simulink model "MON_sl_after_harness"  (R2016a)
settings: Solver=FixedStepDiscrete  StartTime=0  StopTime=0.01  FixedStep=0.01  RelTol=1e-3
undefined symbols (not defined in the file or in its folder): dt, sigbuilder_block
libraries: simulink x1
settings Model: SldvGeneratedHarnessModel=TestUnitModel=MON_sl_after|  MBDTemplateVer=1.1  ModelType=Feature  LastModifiedBy=jdbackes
settings DataIOCC: LimitDataPoints=on  SaveFormat=StructureWithTime
settings OptimizationCC: BlockReduction=off  ExpressionFolding=off
settings DebuggingCC: InheritedTsInSrcMsg=none  AllowSymbolicDim=off
settings ModelReferenceCC: PropagateSignalLabelsOutOfModel=off
settings RTWCC: Description=Generic Real-Time Target
settings GRTTargetCC: GeneratePreprocessorConditionals=Use local settings
settings ConfigComp: DVMode=PropertyProving  DVTestSuiteOptimization=CombinedObjectives (Nonlinear Extended)  DVAssertions=EnableAll  DVProofAssumptions=EnableAll  DVDisplayReport=off

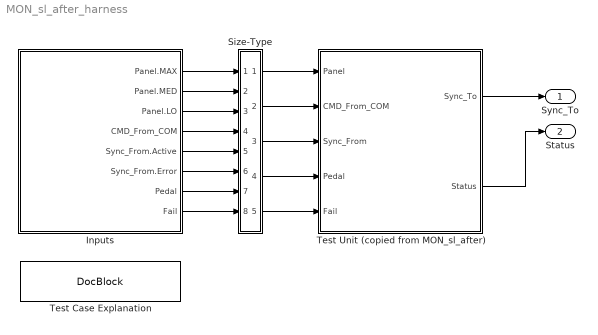
== system MON_sl_after_harness ==
  Inputs : Subsystem  Tag=STV Subsys  LoadFcn=sigbuilder_block('load',[50 50 520 400 ]);  StartFcn=sigbuilder_block('start');  StopFcn=sigbuilder_block('stop');  ClipboardFcn=sigbuilder_block('clipboard');  mask(Sigbuilder block){}
      mask init:
      | if ~strcmp(get_param(bdroot(gcb),'SimulationStatus'),'stopped'),tuvar = sigbuilder_block('maskInit'); end
      settings: CopyFcn=sigbuilder_block('copy');  DeleteFcn=sigbuilder_block('delete');  ModelCloseFcn=sigbuilder_block('modelClose');  PreSaveFcn=sigbuilder_block('preSave');  PauseFcn=sigbuilder_block('pause');  ContinueFcn=sigbuilder_block('continue');  NameChangeFcn=sigbuilder_block('namechange');  OpenFcn=sigbuilder_block('open');  CloseFcn=sigbuilder_block('close');
      mask Display: plot(0, 0, 100, 100,[2, 2, 32, 32, 2], [68, 8, 8, 68, 68],[32, 2], [38, 38], [32, 19, 2],[53, 60, 44], [32, 17, 17, 2],[16, 16, 31, 31]);txt = getActiveGroup(gcbh);text(2, 100, txt,'verticalAlignment', 'top');
  Size-Type : Subsystem
  Test Case Explanation : simulink/Model-Wide Utilities/DocBlock  DocumentType=Text
  Test Unit (copied from MON_sl_after) : Subsystem
  Sync_To : Outport  OutDataTypeStr=Bus: SyncMsgImpl  BusOutputAsStruct=on
  Status : Outport  Port=2  OutDataTypeStr=Bus: ChannelStatusImpl  BusOutputAsStruct=on
  wires:
  Inputs/1(Panel.MAX) -> Size-Type/1(In1)
  Inputs/2(Panel.MED) -> Size-Type/2(In2)
  Inputs/3(Panel.LO) -> Size-Type/3(In3)
  Size-Type/1(Out1) -> Test Unit (copied from MON_sl_after)/1(Panel)
  Inputs/4(CMD_From_COM) -> Size-Type/4(In4)
  Size-Type/2(Out2) -> Test Unit (copied from MON_sl_after)/2(CMD_From_COM)
  Inputs/5(Sync_From.Active) -> Size-Type/5(In5)
  Inputs/6(Sync_From.Error) -> Size-Type/6(In6)
  Size-Type/3(Out3) -> Test Unit (copied from MON_sl_after)/3(Sync_From)
  Inputs/7(Pedal) -> Size-Type/7(In7)
  Size-Type/4(Out4) -> Test Unit (copied from MON_sl_after)/4(Pedal)
  Inputs/8(Fail) -> Size-Type/8(In8)
  Size-Type/5(Out5) -> Test Unit (copied from MON_sl_after)/5(Fail)
  Test Unit (copied from MON_sl_after)/1(Sync_To) -> Sync_To/1
  Test Unit (copied from MON_sl_after)/2(Status) -> Status/1

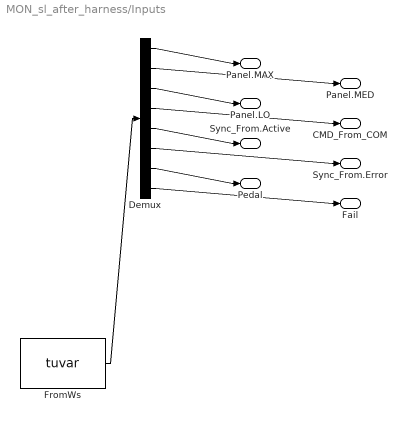
== system MON_sl_after_harness/Inputs ==
  Demux : Demux  Tag=STV Demux  Outputs=8
  FromWs : FromWorkspace  Tag=STV FromWs  VariableName=tuvar  SampleTime=0
      SigBuilderData=|
      | dataSet.timeRange = [0 0.01]
      | dataSet.name = 'Counterexample 1'
      | sbobj.Name = 'Signal Builder'
      | sbobj.Groups.Name = 'Counterexample 1'
      | sbobj.Groups.Signals(1).Name = 'Panel.MAX'
      | sbobj.Groups.Signals(1).XData = [0 0.01]
      | sbobj.Groups.Signals(1).YData = [0 0]
      | sbobj.Groups.Signals(2).Name = 'Panel.MED'
      | sbobj.Groups.Signals(2).XData = [0 0.01]
      | sbobj.Groups.Signals(2).YData = [0 0]
      | sbobj.Groups.Signals(3).Name = 'Panel.LO'
      | sbobj.Groups.Signals(3).XData = [0 0.01]
      | sbobj.Groups.Signals(3).YData = [1 1]
      | sbobj.Groups.Signals(4).Name = 'CMD_From_COM'
      | sbobj.Groups.Signals(4).XData = [0 0.01]
      | sbobj.Groups.Signals(4).YData = [1567609200 1567609200]
      | sbobj.Groups.Signals(5).Name = 'Sync_From.Active'
      | sbobj.Groups.Signals(5).XData = [0 0.01]
      | sbobj.Groups.Signals(5).YData = [1 1]
      | sbobj.Groups.Signals(6).Name = 'Sync_From.Error'
      | sbobj.Groups.Signals(6).XData = [0 0.01]
      | sbobj.Groups.Signals(6).YData = [1 1]
      | sbobj.Groups.Signals(7).Name = 'Pedal'
      | sbobj.Groups.Signals(7).XData = [0 0.01]
      | sbobj.Groups.Signals(7).YData = [1801054272 1801054272]
      | sbobj.Groups.Signals(8).Name = 'Fail'
      | sbobj.Groups.Signals(8).XData = [0 0.01]
      | sbobj.Groups.Signals(8).YData = [0 0]
      | sbobj.Groups.TimeRange = [0 0.01]
  Panel.MAX : Outport  Tag=STV Outport
  Panel.MED : Outport  Tag=STV Outport  Port=2
  Panel.LO : Outport  Tag=STV Outport  Port=3
  CMD_From_COM : Outport  Tag=STV Outport  Port=4
  Sync_From.Active : Outport  Tag=STV Outport  Port=5
  Sync_From.Error : Outport  Tag=STV Outport  Port=6
  Pedal : Outport  Tag=STV Outport  Port=7
  Fail : Outport  Tag=STV Outport  Port=8
  wires:
  FromWs/1 -> Demux/1
  Demux/1 -> Panel.MAX/1
  Demux/2 -> Panel.MED/1
  Demux/3 -> Panel.LO/1
  Demux/4 -> CMD_From_COM/1
  Demux/5 -> Sync_From.Active/1
  Demux/6 -> Sync_From.Error/1
  Demux/7 -> Pedal/1
  Demux/8 -> Fail/1

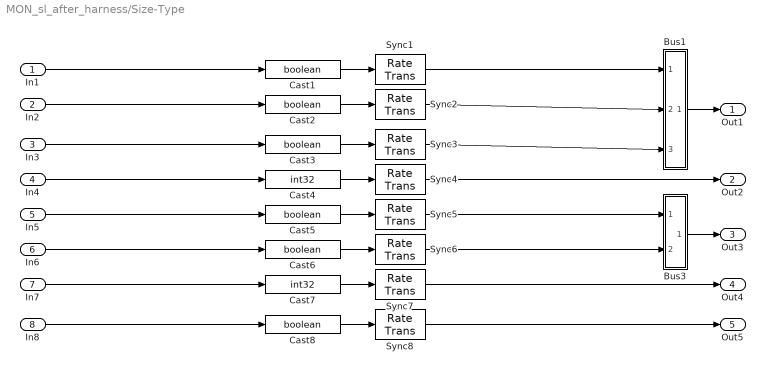
== system MON_sl_after_harness/Size-Type ==
  In1 : Inport
  In2 : Inport  Port=2
  In3 : Inport  Port=3
  In4 : Inport  Port=4
  In5 : Inport  Port=5
  In6 : Inport  Port=6
  In7 : Inport  Port=7
  In8 : Inport  Port=8
  Bus1 : Subsystem
  Bus3 : Subsystem
  Cast{1..3,5..6,8} (6 alike) : DataTypeConversion  OutDataTypeStr=boolean  RndMeth=Nearest  SaturateOnIntegerOverflow=on
  Cast4 : DataTypeConversion  OutDataTypeStr=int32  RndMeth=Nearest  SaturateOnIntegerOverflow=on
  Cast7 : DataTypeConversion  OutDataTypeStr=int32  RndMeth=Nearest  SaturateOnIntegerOverflow=on
  Sync{1..8} (8 alike) : RateTransition  OutPortSampleTime=[0.01,0]
  Out1 : Outport
  Out2 : Outport  Port=2
  Out3 : Outport  Port=3
  Out4 : Outport  Port=4
  Out5 : Outport  Port=5
  wires:
  In1/1 -> Cast1/1
  Cast1/1 -> Sync1/1
  In2/1 -> Cast2/1
  Cast2/1 -> Sync2/1
  In3/1 -> Cast3/1
  Cast3/1 -> Sync3/1
  Sync1/1 -> Bus1/1(Panel(1).MAX)
  Sync2/1 -> Bus1/2(Panel(1).MED)
  Sync3/1 -> Bus1/3(Panel(1).LO)
  Bus1/1(Out) -> Out1/1
  In4/1 -> Cast4/1
  Cast4/1 -> Sync4/1
  Sync4/1 -> Out2/1
  In5/1 -> Cast5/1
  Cast5/1 -> Sync5/1
  In6/1 -> Cast6/1
  Cast6/1 -> Sync6/1
  Sync5/1 -> Bus3/1(Sync_From(1).Active)
  Sync6/1 -> Bus3/2(Sync_From(1).Error)
  Bus3/1(Out) -> Out3/1
  In7/1 -> Cast7/1
  Cast7/1 -> Sync7/1
  Sync7/1 -> Out4/1
  In8/1 -> Cast8/1
  Cast8/1 -> Sync8/1
  Sync8/1 -> Out5/1

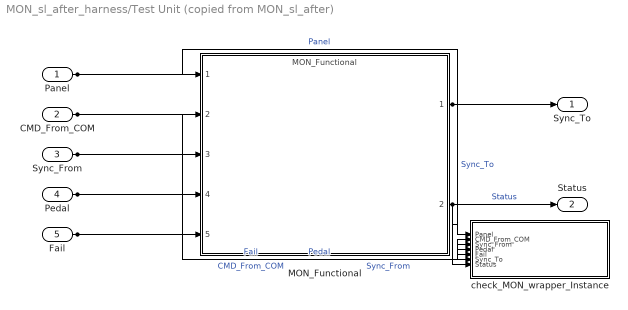
== system MON_sl_after_harness/Test Unit (copied from MON_sl_after) ==
  Panel : Inport  OutDataTypeStr=Bus: PanelMsgImpl  SampleTime=dt  Interpolate=off  BusOutputAsStruct=on
  CMD_From_COM : Inport  Port=2  OutDataTypeStr=int32  SampleTime=dt  Interpolate=off
  Sync_From : Inport  Port=3  OutDataTypeStr=Bus: SyncMsgImpl  SampleTime=dt  Interpolate=off  BusOutputAsStruct=on
  Pedal : Inport  Port=4  OutDataTypeStr=int32  SampleTime=dt  Interpolate=off
  Fail : Inport  Port=5  OutDataTypeStr=boolean  SampleTime=dt  Interpolate=off
  MON_Functional : ModelReference  ModelNameDialog=MON_Functional.slx  SimulationMode=Normal  ModelReferenceVersion=1.2
  check_MON_wrapper_Instance : MATLAB Function  TreatAsAtomicUnit=on  mask(VerificationSubsystem){}
  Sync_To : Outport  OutDataTypeStr=Bus: SyncMsgImpl  BusOutputAsStruct=on
  Status : Outport  Port=2  OutDataTypeStr=Bus: ChannelStatusImpl  BusOutputAsStruct=on
  wires:
  MON_Functional/1 -> check_MON_wrapper_Instance/6(Sync_To), Sync_To/1  "Sync_To"
  MON_Functional/2 -> check_MON_wrapper_Instance/7(Status), Status/1  "Status"
  Panel/1 -> check_MON_wrapper_Instance/1(Panel), MON_Functional/1  "Panel"
  CMD_From_COM/1 -> check_MON_wrapper_Instance/2(CMD_From_COM), MON_Functional/2  "CMD_From_COM"
  Sync_From/1 -> check_MON_wrapper_Instance/3(Sync_From), MON_Functional/3  "Sync_From"
  Pedal/1 -> check_MON_wrapper_Instance/4(Pedal), MON_Functional/4  "Pedal"
  Fail/1 -> check_MON_wrapper_Instance/5(Fail), MON_Functional/5  "Fail"

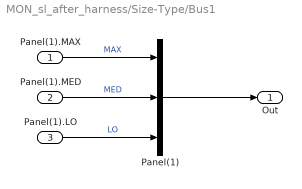
== system MON_sl_after_harness/Size-Type/Bus1 ==
  Panel(1).MAX : Inport
  Panel(1).MED : Inport  Port=2
  Panel(1).LO : Inport  Port=3
  Panel(1) : BusCreator  Inputs=3  OutDataTypeStr=Bus: PanelMsgImpl  NonVirtualBus=on
  Out : Outport
  wires:
  Panel(1).MAX/1 -> Panel(1)/1  "MAX"
  Panel(1).MED/1 -> Panel(1)/2  "MED"
  Panel(1).LO/1 -> Panel(1)/3  "LO"
  Panel(1)/1 -> Out/1

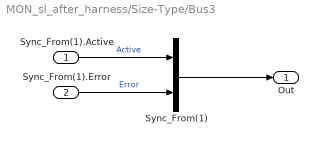
== system MON_sl_after_harness/Size-Type/Bus3 ==
  Sync_From(1).Active : Inport
  Sync_From(1).Error : Inport  Port=2
  Sync_From(1) : BusCreator  Inputs=2  OutDataTypeStr=Bus: SyncMsgImpl  NonVirtualBus=on
  Out : Outport
  wires:
  Sync_From(1).Active/1 -> Sync_From(1)/1  "Active"
  Sync_From(1).Error/1 -> Sync_From(1)/2  "Error"
  Sync_From(1)/1 -> Out/1

== matlab function MON_sl_after_harness/Test Unit (copied from MON_sl_after)/check_MON_wrapper_Instance ==
  data: Panel input; CMD_From_COM input; Sync_From input; Pedal input; Fail input; Sync_To input; Status input
function check_MON_wrapper_Instance(Panel, CMD_From_COM, Sync_From, Pedal, Fail, Sync_To, Status)

persistent pre_c_Agree_Nodes__Duration_0
persistent pre_p_Agree_Nodes__Rise_2_Agree_Nodes__Brake_Mode_0
persistent pre_mode_Agree_Nodes__Brake_Mode_0
persistent pre_Active
persistent first_time
persistent pre_p_Agree_Nodes__Rise_0_Agree_Nodes__Brake_Mode_0
persistent pre_p_Agree_Nodes__Rise_1_Agree_Nodes__Brake_Mode_0
persistent pre_r_Agree_Nodes__Latch_0

Primary_Side = false;
max_Agree_Nodes__Brake_Mode_0 = Panel.MAX;
p_Agree_Nodes__Rise_2_Agree_Nodes__Brake_Mode_0 = max_Agree_Nodes__Brake_Mode_0;

if isempty(pre_p_Agree_Nodes__Rise_2_Agree_Nodes__Brake_Mode_0)
	pre_p_Agree_Nodes__Rise_2_Agree_Nodes__Brake_Mode_0 = (false);
end


if isempty(first_time)
	first_time = true;
end

r_Agree_Nodes__Rise_2_Agree_Nodes__Brake_Mode_0 = arrowFunction(first_time,false, (not(pre_p_Agree_Nodes__Rise_2_Agree_Nodes__Brake_Mode_0) && p_Agree_Nodes__Rise_2_Agree_Nodes__Brake_Mode_0));
lo_Agree_Nodes__Brake_Mode_0 = Panel.LO;
p_Agree_Nodes__Rise_0_Agree_Nodes__Brake_Mode_0 = lo_Agree_Nodes__Brake_Mode_0;

if isempty(pre_p_Agree_Nodes__Rise_0_Agree_Nodes__Brake_Mode_0)
	pre_p_Agree_Nodes__Rise_0_Agree_Nodes__Brake_Mode_0 = (false);
end

r_Agree_Nodes__Rise_0_Agree_Nodes__Brake_Mode_0 = arrowFunction(first_time,false, (not(pre_p_Agree_Nodes__Rise_0_Agree_Nodes__Brake_Mode_0) && p_Agree_Nodes__Rise_0_Agree_Nodes__Brake_Mode_0));
med_Agree_Nodes__Brake_Mode_0 = Panel.MED;
p_Agree_Nodes__Rise_1_Agree_Nodes__Brake_Mode_0 = med_Agree_Nodes__Brake_Mode_0;

if isempty(pre_p_Agree_Nodes__Rise_1_Agree_Nodes__Brake_Mode_0)
	pre_p_Agree_Nodes__Rise_1_Agree_Nodes__Brake_Mode_0 = (false);
end

r_Agree_Nodes__Rise_1_Agree_Nodes__Brake_Mode_0 = arrowFunction(first_time,false, (not(pre_p_Agree_Nodes__Rise_1_Agree_Nodes__Brake_Mode_0) && p_Agree_Nodes__Rise_1_Agree_Nodes__Brake_Mode_0));

if isempty(pre_mode_Agree_Nodes__Brake_Mode_0)
	pre_mode_Agree_Nodes__Brake_Mode_0 = int32(0);
end

r_Agree_Nodes__Brake_Mode_0 = arrowFunction(first_time,int32(1), ifFunction((isequal(pre_mode_Agree_Nodes__Brake_Mode_0, int32(2)) && r_Agree_Nodes__Rise_0_Agree_Nodes__Brake_Mode_0), int32(1), ifFunction((isequal(pre_mode_Agree_Nodes__Brake_Mode_0, int32(3)) && r_Agree_Nodes__Rise_1_Agree_Nodes__Brake_Mode_0), int32(1), ifFunction((isequal(pre_mode_Agree_Nodes__Brake_Mode_0, int32(4)) && r_Agree_Nodes__Rise_2_Agree_Nodes__Brake_Mode_0), int32(1), ifFunction(((pre_mode_Agree_Nodes__Brake_Mode_0 ~= int32(2)) && r_Agree_Nodes__Rise_0_Agree_Nodes__Brake_Mode_0), int32(2), ifFunction(((pre_mode_Agree_Nodes__Brake_Mode_0 ~= int32(3)) && r_Agree_Nodes__Rise_1_Agree_Nodes__Brake_Mode_0), int32(3), ifFunction(((pre_mode_Agree_Nodes__Brake_Mode_0 ~= int32(4)) && r_Agree_Nodes__Rise_2_Agree_Nodes__Brake_Mode_0), int32(4), pre_mode_Agree_Nodes__Brake_Mode_0)))))));
Mode = r_Agree_Nodes__Brake_Mode_0;
p_Agree_Nodes__Duration_0 = not(isequal(Status.Cmd, CMD_From_COM));
b_Agree_Nodes__b2i_0_Agree_Nodes__Duration_0 = p_Agree_Nodes__Duration_0;
i_Agree_Nodes__b2i_0_Agree_Nodes__Duration_0 = ifFunction(b_Agree_Nodes__b2i_0_Agree_Nodes__Duration_0, int32(1), int32(0));

if isempty(pre_c_Agree_Nodes__Duration_0)
	pre_c_Agree_Nodes__Duration_0 = int32(0);
end

c_Agree_Nodes__Duration_0 = arrowFunction(first_time,i_Agree_Nodes__b2i_0_Agree_Nodes__Duration_0, ifFunction(p_Agree_Nodes__Duration_0, (pre_c_Agree_Nodes__Duration_0 + int32(1)), int32(0)));
p_Agree_Nodes__Latch_0 = (c_Agree_Nodes__Duration_0 > int32(15));

if isempty(pre_r_Agree_Nodes__Latch_0)
	pre_r_Agree_Nodes__Latch_0 = (false);
end

r_Agree_Nodes__Latch_0 = arrowFunction(first_time,p_Agree_Nodes__Latch_0, (p_Agree_Nodes__Latch_0 || pre_r_Agree_Nodes__Latch_0));
Error = r_Agree_Nodes__Latch_0;

if isempty(pre_Active)
	pre_Active = (false);
end

Active = arrowFunction(first_time,not(Sync_From.Active), ifFunction(Error, false, ifFunction((((pre_Active && Sync_From.Active) && not(Sync_From.Error)) && not(Primary_Side)), false, ifFunction((not(pre_Active) && (not(Sync_From.Active) || Sync_From.Error)), true, pre_Active))));
pedal_Agree_Nodes__Brake_Cmd_0 = Pedal;
mode_Agree_Nodes__Brake_Cmd_0 = Mode;
r_Agree_Nodes__Brake_Cmd_0 = ifFunction(isequal(mode_Agree_Nodes__Brake_Cmd_0, int32(2)), int32(170), ifFunction(isequal(mode_Agree_Nodes__Brake_Cmd_0, int32(3)), int32(340), ifFunction(isequal(mode_Agree_Nodes__Brake_Cmd_0, int32(4)), int32(510), pedal_Agree_Nodes__Brake_Cmd_0)));
GUARANTEE0 = impliesFunction(not(Fail), isequal(Status.Cmd, r_Agree_Nodes__Brake_Cmd_0));
GUARANTEE1 = ~isequal(Status.Error, Error);
GUARANTEE2 = isequal(Sync_To.Error, Error);
GUARANTEE3 = isequal(Status.Active, Active);
GUARANTEE4 = isequal(Sync_To.Active, Active);
mode_Agree_Nodes__Brake_Mode_0 = Mode;
nodeLemma0_Agree_Nodes__Duration_0 = (c_Agree_Nodes__Duration_0 >= int32(0));
pre_c_Agree_Nodes__Duration_0 = c_Agree_Nodes__Duration_0;
pre_p_Agree_Nodes__Rise_2_Agree_Nodes__Brake_Mode_0 = p_Agree_Nodes__Rise_2_Agree_Nodes__Brake_Mode_0;
pre_mode_Agree_Nodes__Brake_Mode_0 = mode_Agree_Nodes__Brake_Mode_0;
pre_Active = Active;
first_time = false;
pre_p_Agree_Nodes__Rise_0_Agree_Nodes__Brake_Mode_0 = p_Agree_Nodes__Rise_0_Agree_Nodes__Brake_Mode_0;
pre_p_Agree_Nodes__Rise_1_Agree_Nodes__Brake_Mode_0 = p_Agree_Nodes__Rise_1_Agree_Nodes__Brake_Mode_0;
pre_r_Agree_Nodes__Latch_0 = r_Agree_Nodes__Latch_0;

sldv.prove(GUARANTEE0)

sldv.prove(GUARANTEE1)

sldv.prove(GUARANTEE2)

sldv.prove(GUARANTEE3)

sldv.prove(GUARANTEE4)

sldv.prove(nodeLemma0_Agree_Nodes__Duration_0)

end

function output = ifFunction(cond, ifBranch, elseBranch)
if (cond)
	output = ifBranch;
else
	output = elseBranch;
end
end

function output = arrowFunction(first_time, left, right)
if (first_time)
	output = left;
else
	output = right;
end
end

function output = impliesFunction(left, right)
	output = (not(left) || right);
end
